simulink model "PIDdiscret_01"  (Simulink 8.5)
settings: Solver=ode45  StartTime=0.0  StopTime=7  FixedStep=0.001  RelTol=1e-3
values from neighbouring files (symbols this model uses):
  K = (y_real(end) - y_real(1))/(input.signals.values(end) - 0)    [ctr.m]
  L = 1.5*(t1_28 - (t2_63/3))    [ctr.m]
  T = 1.5*(t2_63 - t1_28)    [ctr.m]
settings Model: Creator=guima  LastModifiedBy=guima
settings DataIOCC: SignalLoggingSaveFormat=Dataset
settings OptimizationCC: ExpressionDepthLimit=128
settings DebuggingCC: UnderspecifiedInitializationDetection=Simplified  MergeDetectMultiDrivingBlocksExec=error  FcnCallInpInsideContextMsg=EnableAllAsError  StateNameClashWarn=none
settings GRTTargetCC: CombineOutputUpdateFcns=on  GRTInterface=off

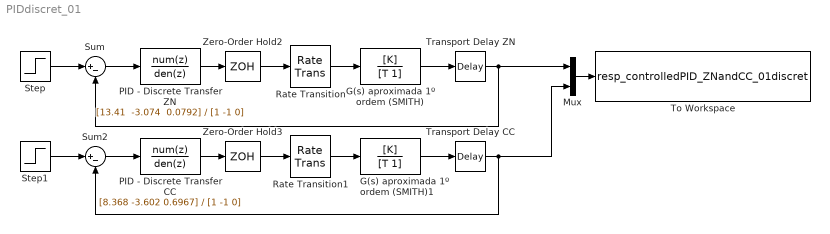
== system PIDdiscret_01 ==
  G(s) aproximada 1º ordem (SMITH) : TransferFcn  Numerator=[K]  Denominator=[T 1]
  G(s) aproximada 1º ordem (SMITH)1 : TransferFcn  Numerator=[K]  Denominator=[T 1]
  Mux : Mux  Inputs=2
  PID - Discrete Transfer CC : DiscreteTransferFcn  Numerator=[8.368 -3.602 0.6967]  Denominator=[1 -1 0]  SampleTime=0.1
  PID - Discrete Transfer ZN : DiscreteTransferFcn  Numerator="[13.41  -3.074  0.0792]"  Denominator=[1 -1 0]  SampleTime=0.1  DenCoefDataTypeStr=int8
  Rate Transition : RateTransition
  Rate Transition1 : RateTransition
  Step : Step  Time=0  SampleTime=0.1
  Step1 : Step  Time=0  SampleTime=0.1
  Sum : Sum  Inputs=|+-
  Sum2 : Sum  Inputs=|+-
  To Workspace : ToWorkspace  VariableName=resp_controlledPID_ZNandCC_01discret  SaveFormat=Structure With Time  SampleTime=-1
  Transport Delay CC : TransportDelay  DelayTime=L
  Transport Delay ZN : TransportDelay  DelayTime=L
  Zero-Order Hold2 : ZeroOrderHold  SampleTime=0.1
  Zero-Order Hold3 : ZeroOrderHold  SampleTime=0.1
  wires:
  Step/1 -> Sum/1
  PID - Discrete Transfer ZN/1 -> Zero-Order Hold2/1
  G(s) aproximada 1º ordem (SMITH)/1 -> Transport Delay ZN/1
  Transport Delay ZN/1 -> Mux/1, Sum/2
  Step1/1 -> Sum2/1
  G(s) aproximada 1º ordem (SMITH)1/1 -> Transport Delay CC/1
  Transport Delay CC/1 -> Sum2/2, Mux/2
  Mux/1 -> To Workspace/1
  PID - Discrete Transfer CC/1 -> Zero-Order Hold3/1
  Sum2/1 -> PID - Discrete Transfer CC/1
  Sum/1 -> PID - Discrete Transfer ZN/1
  Zero-Order Hold2/1 -> Rate Transition/1
  Zero-Order Hold3/1 -> Rate Transition1/1
  Rate Transition/1 -> G(s) aproximada 1º ordem (SMITH)/1
  Rate Transition1/1 -> G(s) aproximada 1º ordem (SMITH)1/1
